simulink model "Three_Band_EQ_Model"  (R2012b)
settings: Solver=FixedStepDiscrete  StartTime=0.0  StopTime=600  RelTol=1e-3
undefined symbols (not defined in the file or in its folder): A1, A2, A3, B1, B2, B3, dfilt
libraries: dsparch4 x3, simulink x3, dspvision x1, dspsnks4 x1
settings Model: Creator=mark  LastModifiedBy=mark
settings DebuggingCC: SolverPrmCheckMsg=none

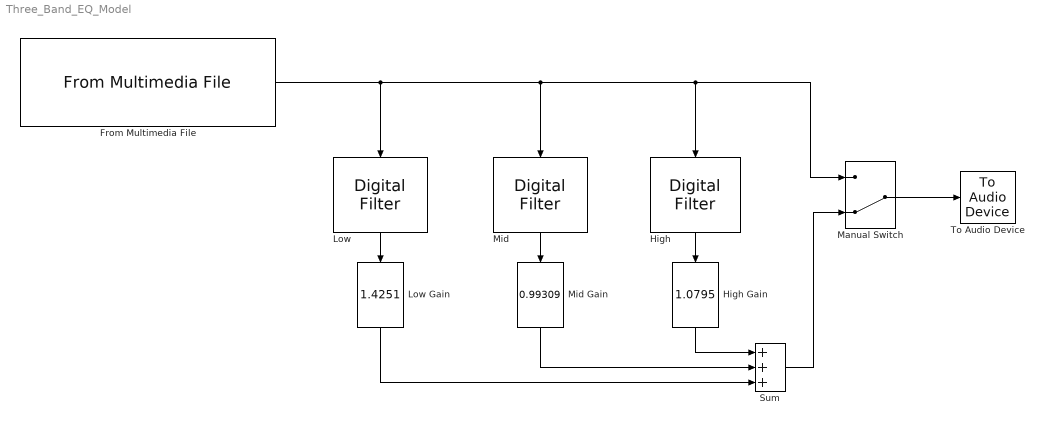
== system Three_Band_EQ_Model ==
  From Multimedia File : dspvision/From Multimedia File  inputFilename=/Users/mark/Music/iTunes/iTunes Music/Basia/Clear Horizon - The Best of Basia/11 An Olive Tree.m4a  loop=on  numPlays=inf  outputStreams=Audio only  videoDataType=single  audioDataType=double  inheritSampleTime=on  userDefinedSampleTime=1/30  noAudioOutput=off  isIntensityVideo=off  fourcc=RGB  colorVideoFormat=Separate color signals  outputEOF=off  dataOrg=Column-major  audioFrameSize=1024  computeAudioFrameSize=off  outSamplingMode=Frame based
  "High  " : dsparch4/Digital Filter  TypePopup=IIR (poles & zeros)  IIRFiltStruct=Direct form II transposed  AllPoleFiltStruct=Direct form  FIRFiltStruct=Direct form  CoeffSource=Specify via dialog  NumCoeffs=[B3]  DenCoeffs=[A3]  BiQuadCoeffs=[1 0.3 0.4 1 0.1 0.2]  LatticeCoeffs=[0.2 0.4]  denIgnore=on  FiltPerSampPopup=One filter per frame  IC=0  ICnum=0  ICden=0  roundingMode=Floor  overflowMode=off  ScaleValues=1  scaleValueFracLength=14  stageInFracLength=15  stageOutFracLength=15  FilterSource=Specify via dialog  dfiltObjectName=dfilt.dffir([1 2 1])  InputProcessing=Columns as channels (frame based)
  "High Gain  " : simulink/Math Operations/Slider Gain  low=0.25  gain=1.0795  high=4
  "Low  " : dsparch4/Digital Filter  TypePopup=IIR (poles & zeros)  IIRFiltStruct=Direct form II transposed  AllPoleFiltStruct=Direct form  FIRFiltStruct=Direct form  CoeffSource=Specify via dialog  NumCoeffs=[B1 ]  DenCoeffs=[A1]  BiQuadCoeffs=[1 0.3 0.4 1 0.1 0.2]  LatticeCoeffs=[0.2 0.4]  denIgnore=on  FiltPerSampPopup=One filter per frame  IC=0  ICnum=0  ICden=0  roundingMode=Floor  overflowMode=off  ScaleValues=1  scaleValueFracLength=14  stageInFracLength=15  stageOutFracLength=15  FilterSource=Specify via dialog  dfiltObjectName=dfilt.dffir([1 2 1])  InputProcessing=Columns as channels (frame based)
  "Low Gain  " : simulink/Math Operations/Slider Gain  low=0.25  gain=1.4251  high=4
  Manual Switch : ManualSwitch  CurrentSetting=0
  "Mid  " : dsparch4/Digital Filter  TypePopup=IIR (poles & zeros)  IIRFiltStruct=Direct form II transposed  AllPoleFiltStruct=Direct form  FIRFiltStruct=Direct form  CoeffSource=Specify via dialog  NumCoeffs=[B2]  DenCoeffs=[A2]  BiQuadCoeffs=[1 0.3 0.4 1 0.1 0.2]  LatticeCoeffs=[0.2 0.4]  denIgnore=on  FiltPerSampPopup=One filter per frame  IC=0  ICnum=0  ICden=0  roundingMode=Floor  overflowMode=off  ScaleValues=1  scaleValueFracLength=14  stageInFracLength=15  stageOutFracLength=15  FilterSource=Specify via dialog  dfiltObjectName=dfilt.dffir([1 2 1])  InputProcessing=Columns as channels (frame based)
  "Mid Gain  " : simulink/Math Operations/Slider Gain  low=0.25  gain=0.99309  high=4
  Sum : Sum  Inputs=+++
  To Audio Device : dspsnks4/To Audio Device  deviceName=Built-in Output  inheritSampleRate=on  sampleRate=44100  deviceDatatype=Determine from input data type  autoBufferSize=on  bufferSize=4096  queueDuration=1.0
  wires:
  "Mid  "/1 -> "Mid Gain  "/1
  "Low  "/1 -> "Low Gain  "/1
  "High  "/1 -> "High Gain  "/1
  "High Gain  "/1 -> Sum/1
  Manual Switch/1 -> To Audio Device/1
  Sum/1 -> Manual Switch/2
  From Multimedia File/1 -> "Low  "/1, "Mid  "/1, Manual Switch/1, "High  "/1
  "Mid Gain  "/1 -> Sum/2
  "Low Gain  "/1 -> Sum/3
